simulink model "differential_equation"  (R2018b)
settings: Solver=ode5  StartTime=0.0  StopTime=10.0  RelTol=1e-3
settings Model: Creator=marwan  LastModifiedBy=marwan

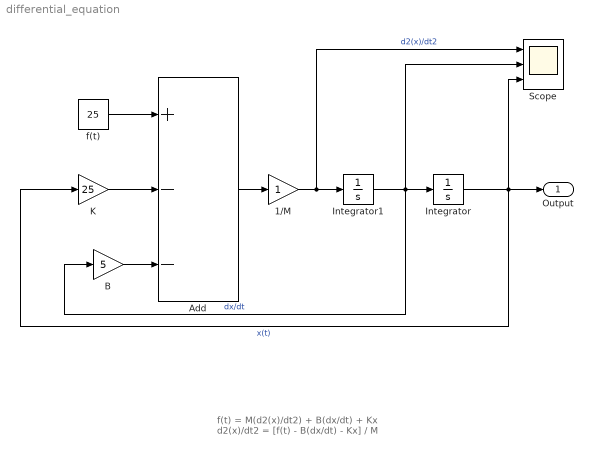
== system differential_equation ==
  note: f(t) = M(d2(x)/dt2) + B(dx/dt) + Kx
      | d2(x)/dt2 = [f(t) - B(dx/dt) - Kx] / M
  1/M : Gain
  Add : Sum  Inputs=+--
  B : Gain  Gain=5
  Integrator : Integrator
  Integrator1 : Integrator
  K : Gain  Gain=25
  Scope : Scope  NumInputPorts=3
  f(t) : Constant  Value=25
  Output : Outport
  wires:
  Integrator/1 -> Scope/3, K/1, Output/1  "x(t)"
  Integrator1/1 -> Scope/2, B/1, Integrator/1  "dx/dt"
  f(t)/1 -> Add/1
  K/1 -> Add/2
  Add/1 -> 1/M/1
  B/1 -> Add/3
  1/M/1 -> Scope/1, Integrator1/1  "d2(x)/dt2"
